simulink model "HEV_ECMS"  (Simulink 9.2)
settings: Solver=FixedStepDiscrete  StartTime=0.0  StopTime=1220  FixedStep=data.dt  RelTol=1e-3  EnableMultiTasking=on
InitFcn:
  | init_HEV_ECMS
StopFcn:
  | if t(end)==str2num(get_param(char(bdroot(gcb)),'StopTime'))
  | msgbox('Simulation completed')
  | else
  | msgbox('Simulation aborted due to limitation in one of the components','','error')
  | end
undefined symbols (not defined in the file or in its folder): data, DiscIntNeverNeededParam, parallelhybrid_ECMS
libraries: simulink x5, qss_tb_library x3
settings Model: Creator=oberg  LastModifiedBy=Mattias  ExtModeAutoUpdateStatusClock=off
settings OptimizationCC: ExpressionDepthLimit=2147483647  InitFltsAndDblsToZero=on
settings DebuggingCC: SaveWithParameterizedLinksMsg=none  SignalResolutionControl=TryResolveAllWithWarning  SolverPrmCheckMsg=warning  MultiTaskDSMMsg=warning  MultiTaskCondExecSysMsg=none
settings GRTTargetCC: TargetFcnLib=ansi_tfl_tmw.mat
settings ConfigComp: CovSFcnEnable=off

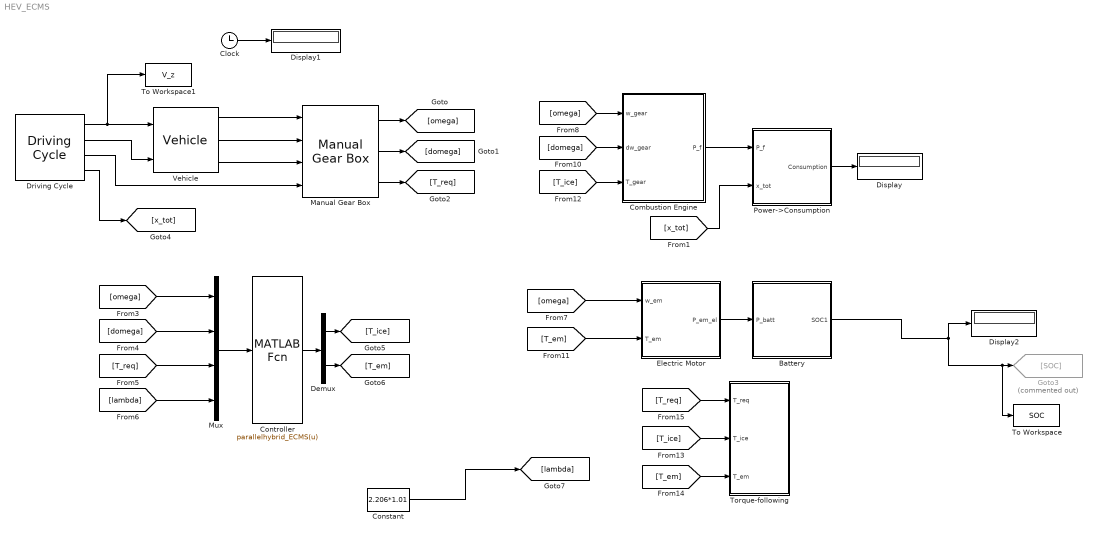
== system HEV_ECMS ==
  Battery : Subsystem  mask{U_oc=data.Uoc, R_i=data.Ri, Q_0=data.Q, SOC_0=0.5, I_max=data.Imax}
      mask prompts: U_oc "Open-Circuit Voltage [V]"; R_i "Inner Resistance [Ohm]"; Q_0 "Capacity [Ah]"; SOC_0 "Initial SOC [-]"; I_max "Max current [I]"
  Clock : Clock
  Combustion Engine : Subsystem
  Constant : Constant  Value=2.206*1.01
  Controller : MATLABFcn  MATLABFcn=parallelhybrid_ECMS(u)
  Demux : Demux  Outputs=2
  Display : Display
  Display1 : Display
  Display2 : Display
  Driving Cycle : qss_tb_library/Driving Cycle/Driving Cycle  Tag=cycle  cyclenr=Europe: NEDC  stepsize=1  autostop=on
  Electric Motor : Subsystem
  Goto3 : Goto  Commented=on  GotoTag=SOC
  Manual Gear Box : qss_tb_library/Gear System/Manual Gear Box  Tag=transmission  i_1=13.0529  i_2=8.1595  i_3=5.6651  i_4=4.2555  i_5=3.2623  i_diff=1  e_GT=0.98  P_GT0=300  w_wheel_min=1
  Mux : Mux
  Power->Consumption : Subsystem  mask{Hlhv=data.Hlhv, rho_f=data.rho_f}
      mask prompts: Hlhv "Lower Heating Value"; rho_f "Density [kg/m^3]"
  To Workspace : ToWorkspace  VariableName=SOC  SaveFormat=Timeseries  SampleTime=-1
  To Workspace1 : ToWorkspace  VariableName=V_z  SaveFormat=Timeseries  SampleTime=-1
  Torque-following : Subsystem
  Vehicle : qss_tb_library/Vehicle/Vehicle  Tag=vehicle  m_f=1500  mt2m_f=0.45  A_f=2.31  r_wheel=0.3  cw=0.32  mu=0.015
  wires:
  Power->Consumption/1(Consumption) -> Display/1
  Combustion Engine/1(P_f) -> Power->Consumption/1(P_f)
  Driving Cycle/1 -> To Workspace1/1, Vehicle/1
  Driving Cycle/2 -> Vehicle/2
  Driving Cycle/3 -> Manual Gear Box/4
  Vehicle/1 -> Manual Gear Box/1
  Vehicle/2 -> Manual Gear Box/2
  Vehicle/3 -> Manual Gear Box/3
  Clock/1 -> Display1/1
  Manual Gear Box/1 -> [omega]
  Manual Gear Box/2 -> [domega]
  Manual Gear Box/3 -> [T_req]
  [x_tot] -> Power->Consumption/2(x_tot)
  Electric Motor/1(P_em_el) -> Battery/1(P_batt)
  Mux/1 -> Controller/1
  [lambda] -> Mux/4
  [omega] -> Electric Motor/1(w_em)
  [omega] -> Combustion Engine/1(w_gear)
  [domega] -> Combustion Engine/2(dw_gear)
  Controller/1 -> Demux/1
  Demux/1 -> [T_ice]
  [T_em] -> Electric Motor/2(T_em)
  [T_ice] -> Combustion Engine/3(T_gear)
  Driving Cycle/4 -> [x_tot]
  Battery/1(SOC1) -> Display2/1, To Workspace/1, Goto3/1
  [T_ice] -> Torque-following/2("T_ice ")
  [T_em] -> Torque-following/3(T_em)
  [T_req] -> Torque-following/1(T_req)
  Demux/2 -> [T_em]
  [omega] -> Mux/1
  [domega] -> Mux/2
  [T_req] -> Mux/3
  Constant/1 -> [lambda]

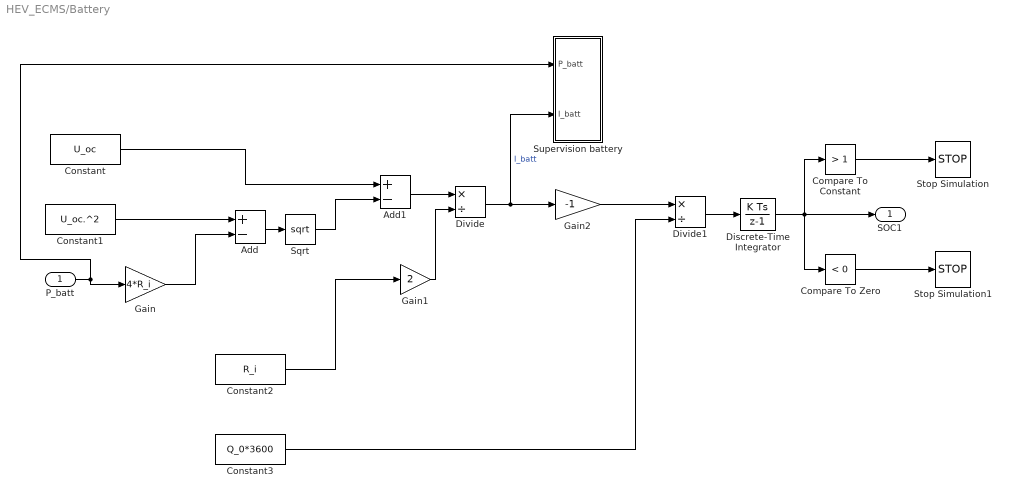
== system HEV_ECMS/Battery ==
  P_batt : Inport
  Add : Sum  Inputs=+-
  Add1 : Sum  Inputs=+-
  Compare To Constant : simulink/Logic and Bit Operations/Compare To Constant  relop=>  const=1  OutDataTypeStr=boolean
  Compare To Zero : simulink/Logic and Bit Operations/Compare To Zero  relop=<  OutDataTypeStr=boolean
  Constant : Constant  Value=U_oc
  Constant1 : Constant  Value=U_oc.^2
  Constant2 : Constant  Value=R_i
  Constant3 : Constant  Value=Q_0*3600
  Discrete-Time Integrator : DiscreteIntegrator  InitialCondition=SOC_0  SampleTime=-1  ICPrevOutput=DiscIntNeverNeededParam  ICPrevScaledInput=DiscIntNeverNeededParam
  Divide : Product  Inputs=*/
  Divide1 : Product  Inputs=*/
  Gain : Gain  Gain=4*R_i
  Gain1 : Gain  Gain=2
  Gain2 : Gain  Gain=-1
  Sqrt : Sqrt  SaturateOnIntegerOverflow=on
  Stop Simulation : Stop
  Stop Simulation1 : Stop
  Supervision battery : Subsystem  AncestorBlock=qss_tb_library/Energy Buffer/Battery/Battery voltage/Supervision battery
  SOC1 : Outport
  wires:
  P_batt/1 -> Gain/1, Supervision battery/1(P_batt)
  Constant1/1 -> Add/1
  Gain/1 -> Add/2
  Add/1 -> Sqrt/1
  Divide/1 -> Supervision battery/2(I_batt), Gain2/1  "I_batt"
  Divide1/1 -> Discrete-Time Integrator/1
  Sqrt/1 -> Add1/2
  Constant/1 -> Add1/1
  Add1/1 -> Divide/1
  Constant2/1 -> Gain1/1
  Gain1/1 -> Divide/2
  Constant3/1 -> Divide1/2
  Gain2/1 -> Divide1/1
  Discrete-Time Integrator/1 -> Compare To Zero/1, SOC1/1, Compare To Constant/1
  Compare To Zero/1 -> Stop Simulation1/1
  Compare To Constant/1 -> Stop Simulation/1

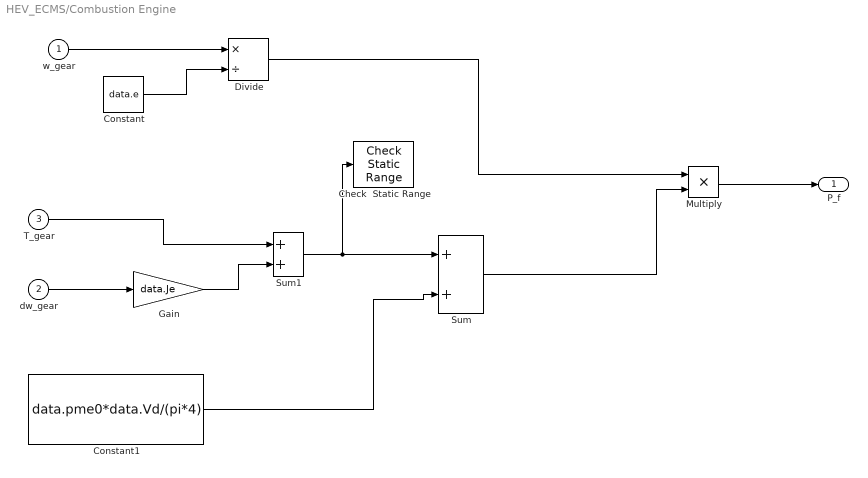
== system HEV_ECMS/Combustion Engine ==
  w_gear : Inport
  dw_gear : Inport  Port=2
  T_gear : Inport  Port=3
  Check  Static Range : simulink/Model Verification/Check  Static Range  Description=0 <= u <= 100  max=100  max_included=on  min=0  min_included=on  enabled=on  stopWhenAssertionFail=on  export=off  icon=graphic
      settings: SourceProductName=Simulink  SourceProductBaseCode=SL
  Constant : Constant  Value=data.e
  Constant1 : Constant  Value=data.pme0*data.Vd/(pi*4)
  Divide : Product  Inputs=*/
  Gain : Gain  Gain=data.Je
  Multiply : Product
  Sum : Sum
  Sum1 : Sum
  P_f : Outport
  wires:
  dw_gear/1 -> Gain/1
  w_gear/1 -> Divide/1
  Constant/1 -> Divide/2
  Multiply/1 -> P_f/1
  Sum/1 -> Multiply/2
  Divide/1 -> Multiply/1
  Constant1/1 -> Sum/2
  Gain/1 -> Sum1/2
  T_gear/1 -> Sum1/1
  Sum1/1 -> Check  Static Range/1, Sum/1

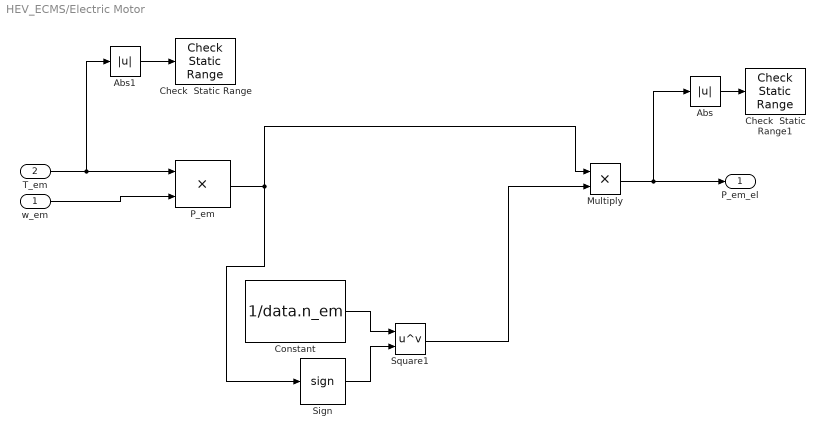
== system HEV_ECMS/Electric Motor ==
  w_em : Inport
  T_em : Inport  Port=2
  Abs : Abs
  Abs1 : Abs
  Check  Static Range : simulink/Model Verification/Check  Static Range  Description=0 <= u <= 100  max=100  max_included=on  min=0  min_included=on  enabled=on  stopWhenAssertionFail=on  export=off  icon=graphic
      settings: SourceProductName=Simulink  SourceProductBaseCode=SL
  Check  Static Range1 : simulink/Model Verification/Check  Static Range  Description=0 <= u <= 100  max=100  max_included=on  min=0  min_included=on  enabled=on  stopWhenAssertionFail=on  export=off  icon=graphic
      settings: SourceProductName=Simulink  SourceProductBaseCode=SL
  Constant : Constant  Value=1/data.n_em
  Multiply : Product
  P_em : Product
  Sign : Signum
  Square1 : Math  Operator=pow  SaturateOnIntegerOverflow=on
  P_em_el : Outport
  wires:
  w_em/1 -> P_em/2
  T_em/1 -> Abs1/1, P_em/1
  P_em/1 -> Sign/1, Multiply/1
  Multiply/1 -> Abs/1, P_em_el/1
  Square1/1 -> Multiply/2
  Constant/1 -> Square1/1
  Sign/1 -> Square1/2
  Abs1/1 -> Check  Static Range/1
  Abs/1 -> Check  Static Range1/1

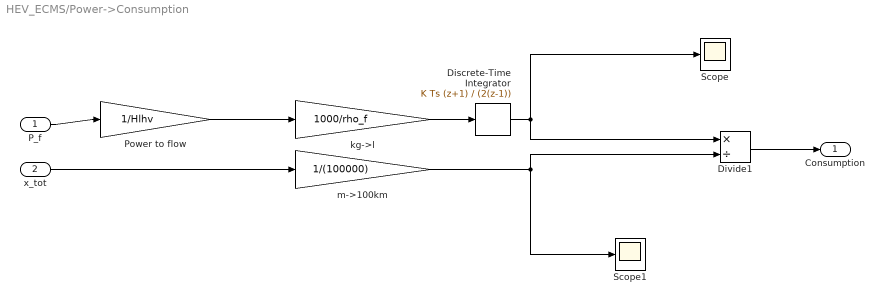
== system HEV_ECMS/Power->Consumption ==
  P_f : Inport
  x_tot : Inport  Port=2
  Discrete-Time Integrator : DiscreteIntegrator  IntegratorMethod=Integration: Trapezoidal  SampleTime=-1  ICPrevOutput=DiscIntNeverNeededParam  ICPrevScaledInput=DiscIntNeverNeededParam
  Divide1 : Product  Inputs=*/
  Power to flow : Gain  Gain=1/Hlhv
  Scope : Scope
  Scope1 : Scope
  kg->l : Gain  Gain=1000/rho_f
  m->100km : Gain  Gain=1/(100000)
  Consumption : Outport
  wires:
  Divide1/1 -> Consumption/1
  P_f/1 -> Power to flow/1
  Power to flow/1 -> kg->l/1
  kg->l/1 -> Discrete-Time Integrator/1
  x_tot/1 -> m->100km/1
  m->100km/1 -> Divide1/2, Scope1/1
  Discrete-Time Integrator/1 -> Divide1/1, Scope/1

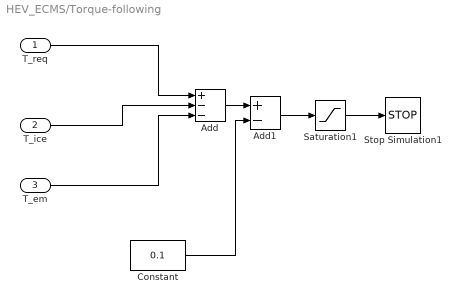
== system HEV_ECMS/Torque-following ==
  T_req : Inport
  "T_ice " : Inport  Port=2
  T_em : Inport  Port=3
  Add : Sum  Inputs=+--
  Add1 : Sum  Inputs=+-
  Constant : Constant  Value=0.1
  Saturation1 : Saturate  UpperLimit=inf  LowerLimit=0
  Stop Simulation1 : Stop
  wires:
  "T_ice "/1 -> Add/2
  T_em/1 -> Add/3
  T_req/1 -> Add/1
  Saturation1/1 -> Stop Simulation1/1
  Add/1 -> Add1/1
  Constant/1 -> Add1/2
  Add1/1 -> Saturation1/1

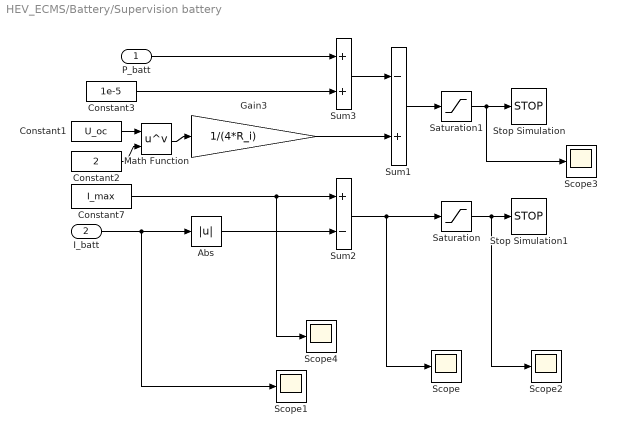
== system HEV_ECMS/Battery/Supervision battery ==
  P_batt : Inport
  I_batt : Inport  Port=2
  Abs : Abs  SaturateOnIntegerOverflow=on
  Constant1 : Constant  Value=U_oc
  Constant2 : Constant  Value=2
  Constant3 : Constant  Value=1e-5
  Constant7 : Constant  Value=I_max
  Gain3 : Gain  Gain=1/(4*R_i)  SaturateOnIntegerOverflow=on  OutDataTypeStr=Inherit: Same as input  ParamDataTypeStr=Inherit: Same as input
  Math Function : Math  Operator=pow  SaturateOnIntegerOverflow=on
  Saturation : Saturate  UpperLimit=0  LowerLimit=-inf
  Saturation1 : Saturate  UpperLimit=0  LowerLimit=-inf
  Scope{,1..4} (5 alike) : Scope
  Stop Simulation : Stop
  Stop Simulation1 : Stop
  Sum1 : Sum  Inputs=-+  SaturateOnIntegerOverflow=on  InputSameDT=on  OutDataTypeStr=Inherit: Same as first input
  Sum2 : Sum  Inputs=+-  SaturateOnIntegerOverflow=on  InputSameDT=on  OutDataTypeStr=Inherit: Same as first input
  Sum3 : Sum  SaturateOnIntegerOverflow=on  InputSameDT=on  OutDataTypeStr=Inherit: Same as first input
  wires:
  Abs/1 -> Sum2/2
  I_batt/1 -> Abs/1, Scope1/1
  Sum2/1 -> Saturation/1, Scope/1
  Constant7/1 -> Sum2/1, Scope4/1
  P_batt/1 -> Sum3/1
  Sum1/1 -> Saturation1/1
  Saturation1/1 -> Stop Simulation/1, Scope3/1
  Saturation/1 -> Stop Simulation1/1, Scope2/1
  Gain3/1 -> Sum1/2
  Sum3/1 -> Sum1/1
  Constant1/1 -> Math Function/1
  Math Function/1 -> Gain3/1
  Constant2/1 -> Math Function/2
  Constant3/1 -> Sum3/2
